simulink model "MotorUNDReifen_Model"  (R2024a)
settings: Solver=VariableStepAuto  StartTime=0.0  StopTime=10.0  RelTol=1e-3
PreLoadFcn:
  | run('Parameter.m')
values from neighbouring files (symbols this model uses):
  A_neu = [0 1 0; 0 A22 A23; 0 A32 A33]    [Parameter.m]
  B_neu = [0; 0; 1/motorinductivity]    [Parameter.m]
  CT_npos = [1 0 0]    [Parameter.m]
  CT_nvel = [0 1 0]    [Parameter.m]
  E_neu = [0; -((m_last/2 + m_Reifen) * g * mue * Reifen_Radius); 0 ]    [Parameter.m]
  Motoruebersetzung = 100    [Model1Sensibilities.m]    (also in Model1numericalPSA.m; Model2Sensibilities.m; Modellvalidierung.m; MotorSens2.m)
  x0_neu = [0; 0.01; 0]    [Parameter.m]
settings Model: Creator=jakob  LastModifiedBy=jakob

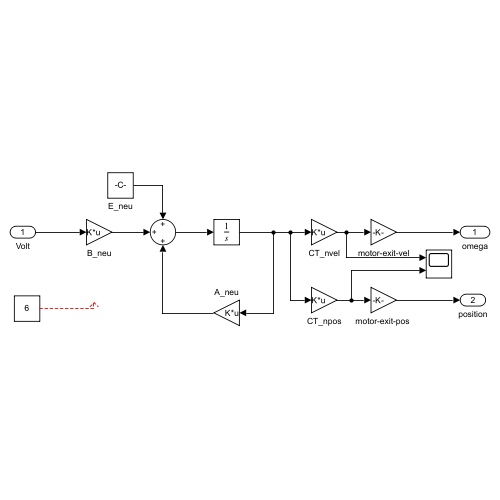
[thumbnail: Simulink's stored preview of the top-level diagram]
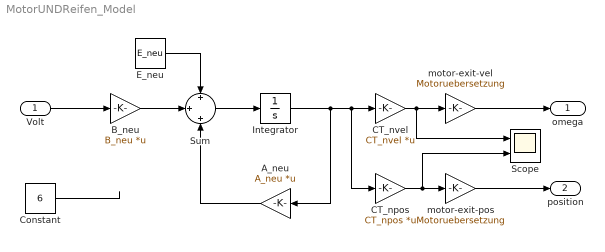
== system MotorUNDReifen_Model ==
  Volt : Inport
  A_neu : Gain  Gain=A_neu  Multiplication=Matrix(K*u)
  B_neu : Gain  Gain=B_neu  Multiplication=Matrix(K*u)
  CT_npos : Gain  Gain=CT_npos  Multiplication=Matrix(K*u)
  CT_nvel : Gain  Gain=CT_nvel  Multiplication=Matrix(K*u)
  Constant : Constant  Value=6
  E_neu : Constant  Value=E_neu
  Integrator : Integrator  InitialCondition=x0_neu
  Scope : Scope  NumInputPorts=2
  Sum : Sum  Inputs=+|+|+
  "motor-exit-pos " : Gain  Gain=Motoruebersetzung
  motor-exit-vel : Gain  Gain=Motoruebersetzung
  omega : Outport
  position : Outport  Port=2
  wires:
  B_neu/1 -> Sum/2
  E_neu/1 -> Sum/1
  Sum/1 -> Integrator/1
  Integrator/1 -> CT_npos/1, CT_nvel/1, A_neu/1
  A_neu/1 -> Sum/3
  CT_nvel/1 -> Scope/1, motor-exit-vel/1
  motor-exit-vel/1 -> omega/1
  CT_npos/1 -> Scope/2, "motor-exit-pos "/1
  "motor-exit-pos "/1 -> position/1
  Constant/1 -> ?
  Volt/1 -> B_neu/1
